simulink model "Experimental_estimation_J"  (R2022b)
settings: Solver=VariableStepAuto  StartTime=0.0  StopTime=10.0  RelTol=1e-3
undefined symbols (not defined in the file or in its folder): Hi, Hw, sens
libraries: arduinolib x5, simulink x1
settings Model: Creator=berti  LastModifiedBy=berti

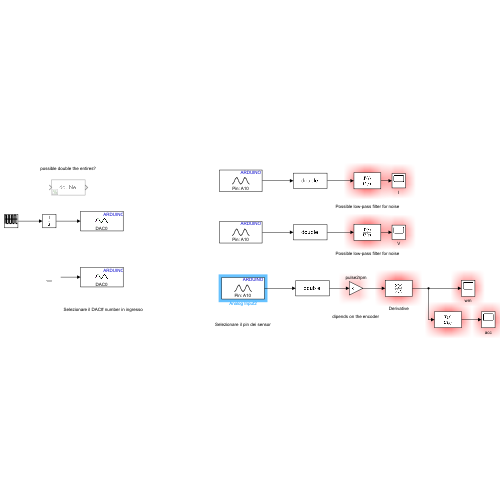
[thumbnail: Simulink's stored preview of the top-level diagram]
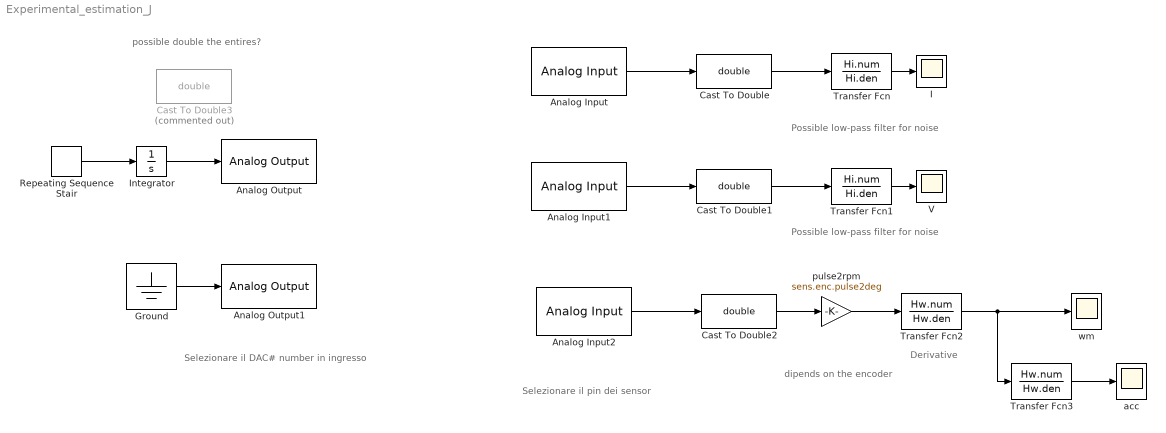
== system Experimental_estimation_J ==
  note: Selezionare il pin dei sensor
  note: Selezionare il DAC# number in ingresso
  note: Derivative
  note: Possible low-pass filter for noise
  note: Possible low-pass filter for noise
  note: dipends on the encoder
  note: possible double the entires?
  Analog Input : arduinolib/Analog Input  pinNumber=10  ReadResultsOnly=off  ConversionTriggerSource=Software  ExternalTriggerType=uint32( 0 )  OutputDataType=uint16  EnableConversionCompleteNotify=off  EnableOuputStatus=off  SampleTime=t  blockPlatform=arduino
  Analog Input1 : arduinolib/Analog Input  pinNumber=10  ReadResultsOnly=off  ConversionTriggerSource=Software  ExternalTriggerType=uint32( 0 )  OutputDataType=uint16  EnableConversionCompleteNotify=off  EnableOuputStatus=off  SampleTime=t  blockPlatform=arduino
  Analog Input2 : arduinolib/Analog Input  pinNumber=10  ReadResultsOnly=off  ConversionTriggerSource=Software  ExternalTriggerType=uint32( 0 )  OutputDataType=uint16  EnableConversionCompleteNotify=off  EnableOuputStatus=off  SampleTime=t  blockPlatform=arduino
  Analog Output : arduinolib/Analog Output  DACpin=DAC0  blockPlatform=arduino
  Analog Output1 : arduinolib/Analog Output  DACpin=DAC0  blockPlatform=arduino
  Cast To Double : DataTypeConversion  OutDataTypeStr=double  SaturateOnIntegerOverflow=off  RndMeth=Floor
  Cast To Double1 : DataTypeConversion  OutDataTypeStr=double  SaturateOnIntegerOverflow=off  RndMeth=Floor
  Cast To Double2 : DataTypeConversion  OutDataTypeStr=double  SaturateOnIntegerOverflow=off  RndMeth=Floor
  Cast To Double3 : DataTypeConversion  Commented=on  OutDataTypeStr=double  SaturateOnIntegerOverflow=off  RndMeth=Floor
  Ground : Ground
  I : Scope
  Integrator : Integrator
  Repeating Sequence Stair : simulink/Sources/Repeating Sequence Stair  OutValues=[1 -1 1 -1 1 -1 1 -1 ].'  tsamp=1  OutMin=[]  OutMax=[]  OutDataTypeStr=double  OutputDataTypeScalingMode=double  OutDataType=fixdt(0,8)  ConRadixGroup=Best Precision: Vector-wise  OutScaling=2^-12
  Transfer Fcn : TransferFcn  Numerator=Hi.num  Denominator=Hi.den
  Transfer Fcn1 : TransferFcn  Numerator=Hi.num  Denominator=Hi.den
  Transfer Fcn2 : TransferFcn  Numerator=Hw.num  Denominator=Hw.den
  Transfer Fcn3 : TransferFcn  Numerator=Hw.num  Denominator=Hw.den
  V : Scope
  acc : Scope
  pulse2rpm : Gain  Gain=sens.enc.pulse2deg
  wm : Scope
  wires:
  Transfer Fcn1/1 -> V/1
  Cast To Double2/1 -> pulse2rpm/1
  Cast To Double1/1 -> Transfer Fcn1/1
  Cast To Double/1 -> Transfer Fcn/1
  Transfer Fcn/1 -> I/1
  Transfer Fcn3/1 -> acc/1
  pulse2rpm/1 -> Transfer Fcn2/1
  Repeating Sequence Stair/1 -> Integrator/1
  Transfer Fcn2/1 -> wm/1, Transfer Fcn3/1
  Analog Input/1 -> Cast To Double/1
  Analog Input2/1 -> Cast To Double2/1
  Analog Input1/1 -> Cast To Double1/1
  Ground/1 -> Analog Output1/1
  Integrator/1 -> Analog Output/1
